simulink model "linear_simulation"  (R2022b)
settings: Solver=FixedStepAuto  StartTime=0.0  StopTime=10.0  FixedStep=1e-4  RelTol=1e-3  EnableMultiTasking=on
values from neighbouring files (symbols this model uses):
  beta = [0.5;2;2;0.5;1]    [Linear_optimal.m]
  delta = 1    [Linear_optimal.m]
  kl1 = sym2poly(kl1)    [Linear_optimal.m]
  kl2 = sym2poly(kl2)    [Linear_optimal.m]
  kn1 = sym2poly(kn1)    [Linear_optimal.m]
  kn2 = sym2poly(kn2)    [Linear_optimal.m]
libraries: simulink x6
settings Model: Creator=sf  LastModifiedBy=sf
settings ModelReferenceCC: EnableRefExpFcnMdlSchedulingChecks=on

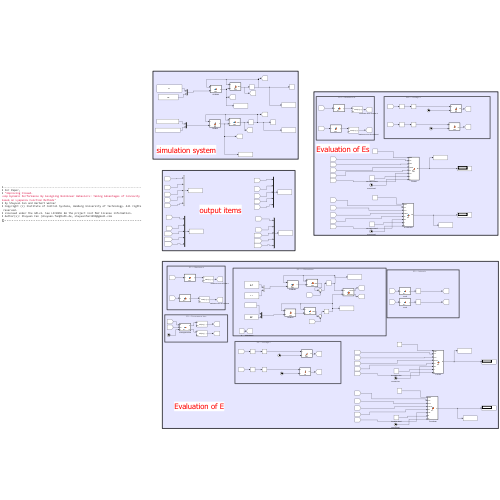
[thumbnail: Simulink's stored preview of the top-level diagram]
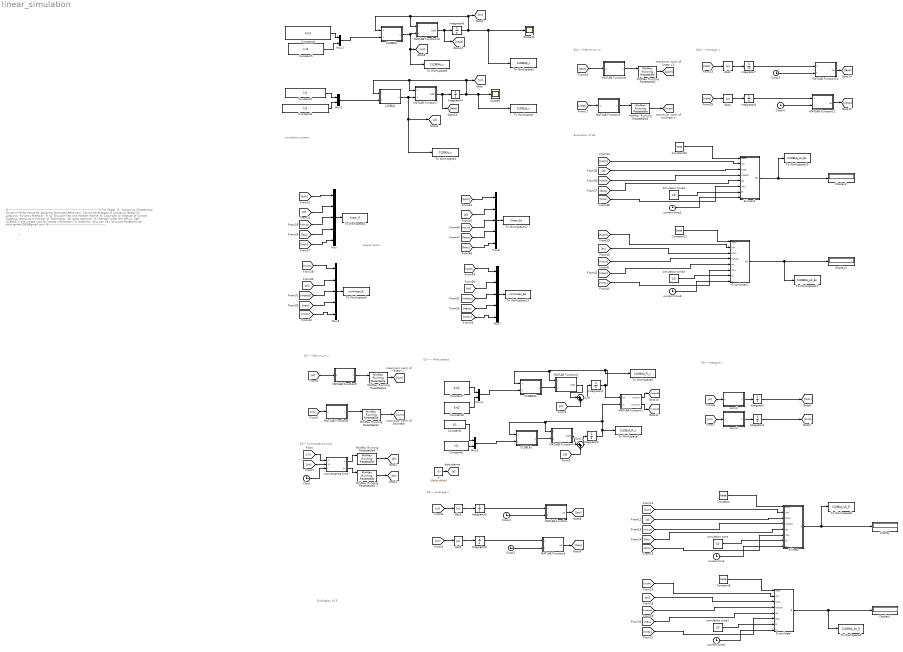
== system linear_simulation ==
  note: )
  note: %-----------------------------------------------------------------------------------------
      | % For Paper,
      | % "Improving Closed-Loop Dynamic Performance By Assigning Nonlinear Behaviors: Taking Advantages of Concavity Based on Lyapunov Function Methods"
      | % by Shuyuan Fan and Herbert Werner
      | % Copyright (c) Institute of Control Systems, Hamburg University of Technology. All rights reserved.
      | % Licensed under the GPLv3. See LICENSE in the project root for license information.
      | % Author(s): Shuyuan Fan (shuyuan.fan@tuhh.de, shuyuanfan1993@gmail.com
      | %---------------------------------------------------------
  note: Evaluation of E
  note: E5-----Integral x
  note: E3-------Robustness
  note: E1-----Maximum u
  note: E2----Convergence time
  note: E4-----everage u
  note: Es1-----Maximum us
  note: Es4-----everage u
  note: Evaluation of Es
  note: simulation system
  note: output items
  Abs{1..4} (4 alike) : Abs  SaturateOnIntegerOverflow=off
  CLDBLA : MATLAB Function  TreatAsAtomicUnit=on
  CLDBLA1 : MATLAB Function  TreatAsAtomicUnit=on
  CLDBNA : MATLAB Function  TreatAsAtomicUnit=on
  CLDBNA1 : MATLAB Function  TreatAsAtomicUnit=on
  Clock{,1..4} (5 alike) : Clock
  Constant{,9..11} (4 alike) : Constant  Value=beta
  Constant1 : Constant  Value=kl1
  Constant2 : Constant  Value=kl1
  Constant3 : Constant  Value=kl2
  Constant4 : Constant  Value=kn1
  Constant5 : Constant  Value=kn2
  Constant6 : Constant  Value=kl2
  Constant7 : Constant  Value=kn1
  Constant8 : Constant  Value=kn2
  Display{,1..3} (4 alike) : Display
  E-linear : MATLAB Function  TreatAsAtomicUnit=on
  E-linear1 : MATLAB Function  TreatAsAtomicUnit=on
  E-nonlinear : MATLAB Function  TreatAsAtomicUnit=on
  E-nonlinear1 : MATLAB Function  TreatAsAtomicUnit=on
  Integrator{,1,5..7,9} (6 alike) : Integrator
  Integrator{2..4,8} (4 alike) : Integrator  InitialCondition=[2;1]
  MATLAB Function : MATLAB Function  TreatAsAtomicUnit=on
  MATLAB Function1 : MATLAB Function  TreatAsAtomicUnit=on
  MATLAB Function10 : MATLAB Function  TreatAsAtomicUnit=on
  MATLAB Function11 : MATLAB Function  TreatAsAtomicUnit=on
  MATLAB Function13 : MATLAB Function  TreatAsAtomicUnit=on
  MATLAB Function2 : MATLAB Function  TreatAsAtomicUnit=on
  MATLAB Function3 : MATLAB Function  TreatAsAtomicUnit=on
  MATLAB Function4 : MATLAB Function  TreatAsAtomicUnit=on
  MATLAB Function5 : MATLAB Function  TreatAsAtomicUnit=on
  MATLAB Function6 : MATLAB Function  TreatAsAtomicUnit=on
  MATLAB Function7 : MATLAB Function  TreatAsAtomicUnit=on
  MATLAB Function8 : MATLAB Function  TreatAsAtomicUnit=on
  MATLAB Function9 : MATLAB Function  TreatAsAtomicUnit=on
  MinMax Running Resettable{1..3,7} (4 alike) : simulink/Math Operations/MinMax Running Resettable  Function=max  vinit=0.0
  MinMax Running Resettable4 : simulink/Math Operations/MinMax Running Resettable  Function=min  vinit=100
  MinMax Running Resettable5 : simulink/Math Operations/MinMax Running Resettable  Function=min  vinit=100
  Mux{,5..7} (4 alike) : Mux  Inputs=5
  Mux{1..4} (4 alike) : Mux  Inputs=2
  Scope11 : Scope
  Scope6 : Scope
  Sum : Sum  Inputs=|++
  Sum1 : Sum  Inputs=|++
  To Workspace : ToWorkspace  VariableName=CLDBLA_x  SaveFormat=Timeseries  SampleTime=-1
  To Workspace1 : ToWorkspace  VariableName=CLDBNA_x  SaveFormat=Timeseries  SampleTime=-1
  To Workspace10 : ToWorkspace  VariableName=CLDBLA_ob_Es  SaveFormat=Timeseries  SampleTime=-1
  To Workspace11 : ToWorkspace  VariableName=CLDBNA_ob_Es  SaveFormat=Timeseries  SampleTime=-1
  To Workspace12 : ToWorkspace  VariableName=linear_Es  SaveFormat=Timeseries  SampleTime=-1
  To Workspace13 : ToWorkspace  VariableName=nonlinear_Es  SaveFormat=Timeseries  SampleTime=-1
  To Workspace2 : ToWorkspace  VariableName=linear_E  SaveFormat=Timeseries  SampleTime=-1
  To Workspace3 : ToWorkspace  VariableName=nonlinear_E  SaveFormat=Timeseries  SampleTime=-1
  To Workspace4 : ToWorkspace  VariableName=CLDBLA_u  SaveFormat=Timeseries  SampleTime=-1
  To Workspace5 : ToWorkspace  VariableName=CLDBNA_u  SaveFormat=Timeseries  SampleTime=-1
  To Workspace6 : ToWorkspace  VariableName=CLDBNA_R_x  SaveFormat=Timeseries  SampleTime=-1
  To Workspace7 : ToWorkspace  VariableName=CLDBLA_R_x  SaveFormat=Timeseries  SampleTime=-1
  To Workspace8 : ToWorkspace  VariableName=CLDBLA_ob_E  SaveFormat=Timeseries  SampleTime=-1
  To Workspace9 : ToWorkspace  VariableName=CLDBNA_ob_E  SaveFormat=Timeseries  SampleTime=-1
  convergence time : MATLAB Function  TreatAsAtomicUnit=on
  current time{,1..3} (4 alike) : Clock
  d : Constant  Value=[delta;delta]
  norm2 : MATLAB Function  TreatAsAtomicUnit=on
  norm3 : MATLAB Function  TreatAsAtomicUnit=on
  simulation time{,1..3} (4 alike) : Constant  Value=10
  wires:
  Constant5/1 -> Mux2/2
  MATLAB Function7/1(xdot) -> [ldot], Integrator4/1
  Constant2/1 -> Mux1/1
  CLDBLA/1(u) -> To Workspace4/1, [ul], MATLAB Function7/2(u)
  Mux1/1 -> CLDBLA/2(k)
  Constant3/1 -> Mux1/2
  Mux2/1 -> CLDBNA/2(k)
  Constant4/1 -> Mux2/1
  MATLAB Function13/1(xdot) -> [ndot], Integrator8/1
  Integrator8/1 -> To Workspace1/1, Scope11/1, [xn], CLDBNA/1(x), MATLAB Function13/1(x)
  MATLAB Function5/1(y) -> MinMax Running Resettable1/1
  CLDBNA/1(u) -> To Workspace5/1, [un], MATLAB Function13/2(u)
  MinMax Running Resettable1/1 -> [lum]
  Clock/1 -> convergence time/3(t)
  Integrator4/1 -> To Workspace/1, Scope6/1, [xl], CLDBLA/1(x), MATLAB Function7/1(x)
  [xl] -> convergence time/1(xl)
  [xn] -> convergence time/2(xn)
  convergence time/1(tl) -> MinMax Running Resettable4/1
  convergence time/2(tn) -> MinMax Running Resettable5/1
  MinMax Running Resettable4/1 -> [tl]
  MinMax Running Resettable5/1 -> [tn]
  MATLAB Function2/1(xdot) -> Sum/1
  Mux4/1 -> CLDBNA1/2(k)
  Constant7/1 -> Mux4/1
  CLDBNA1/1(u) -> MATLAB Function2/2(u)
  CLDBLA1/1(u) -> MATLAB Function4/2(u)
  Constant6/1 -> Mux3/2
  Mux3/1 -> CLDBLA1/2(k)
  Constant8/1 -> Mux4/2
  Integrator3/1 -> MATLAB Function1/1(xn), To Workspace6/1, CLDBNA1/1(x), MATLAB Function2/1(x)
  Constant1/1 -> Mux3/1
  Integrator2/1 -> MATLAB Function1/2(xl), CLDBLA1/1(x), MATLAB Function4/1(x), To Workspace7/1
  MATLAB Function4/1(xdot) -> Sum1/1
  Sum/1 -> Integrator3/1
  Sum1/1 -> Integrator2/1
  d/1 -> [d]
  [d] -> Sum/2
  [d] -> Sum1/2
  [ul] -> MATLAB Function5/1(u)
  [un] -> MATLAB Function6/1(u)
  MinMax Running Resettable7/1 -> [num]
  [xl] -> norm2/1(u)
  norm2/1(y) -> Integrator/1
  Integrator/1 -> [lintx]
  Integrator1/1 -> [nintx]
  norm3/1(y) -> Integrator1/1
  [xn] -> norm3/1(u)
  [un] -> Abs3/1
  [ul] -> Abs2/1
  Abs3/1 -> Integrator6/1
  Abs2/1 -> Integrator5/1
  Integrator5/1 -> MATLAB Function/1(u)
  Clock1/1 -> MATLAB Function/2(t)
  Clock2/1 -> MATLAB Function3/2(t)
  Integrator6/1 -> MATLAB Function3/1(u)
  MATLAB Function/1(ua) -> [lau]
  MATLAB Function3/1(ua) -> [nau]
  MATLAB Function1/1(normxl) -> [lrobust]
  MATLAB Function1/2(normxn) -> [nrobust]
  [lum] -> E-linear/2(um)
  [tl] -> E-linear/3(tcon)
  [lrobust] -> E-linear/4(robust)
  [lau] -> E-linear/5(au)
  [lintx] -> E-linear/6(intx)
  simulation time/1 -> E-linear/7(tf)
  current time/1 -> E-linear/8(tc)
  Constant/1 -> E-linear/1(beta)
  E-linear/1(E) -> To Workspace8/1, Display/1
  [nrobust] -> E-nonlinear/4(robust)
  E-nonlinear/1(E) -> To Workspace9/1, Display1/1
  current time1/1 -> E-nonlinear/8(tc)
  Constant9/1 -> E-nonlinear/1(beta)
  [num] -> E-nonlinear/2(um)
  simulation time1/1 -> E-nonlinear/7(tf)
  [tn] -> E-nonlinear/3(tcon)
  [nintx] -> E-nonlinear/6(intx)
  [nau] -> E-nonlinear/5(au)
  [lum] -> Mux/1
  [tl] -> Mux/2
  [lrobust] -> Mux/3
  [lau] -> Mux/4
  [lintx] -> Mux/5
  Mux/1 -> To Workspace2/1
  Mux5/1 -> To Workspace3/1
  [num] -> Mux5/1
  [tn] -> Mux5/2
  [nrobust] -> Mux5/3
  [nau] -> Mux5/4
  [nintx] -> Mux5/5
  MATLAB Function6/1(y) -> MinMax Running Resettable7/1
  [ndot] -> MATLAB Function9/1(u)
  [ldot] -> MATLAB Function8/1(u)
  MATLAB Function8/1(y) -> MinMax Running Resettable2/1
  MATLAB Function9/1(y) -> MinMax Running Resettable3/1
  MinMax Running Resettable3/1 -> [nusm]
  MinMax Running Resettable2/1 -> [lusm]
  Integrator9/1 -> MATLAB Function11/1(u)
  Clock3/1 -> MATLAB Function10/2(t)
  MATLAB Function11/1(ua) -> [naus]
  [ldot] -> Abs1/1
  Integrator7/1 -> MATLAB Function10/1(u)
  Clock4/1 -> MATLAB Function11/2(t)
  MATLAB Function10/1(ua) -> [laus]
  Abs1/1 -> Integrator7/1
  Abs4/1 -> Integrator9/1
  [ndot] -> Abs4/1
  E-nonlinear1/1(Es) -> To Workspace11/1, Display3/1
  simulation time3/1 -> E-nonlinear1/7(tf)
  [lintx] -> E-linear1/6(intx)
  [lrobust] -> E-linear1/4(robust)
  [naus] -> E-nonlinear1/5(au)
  simulation time2/1 -> E-linear1/7(tf)
  [tl] -> E-linear1/3(tcon)
  [nintx] -> E-nonlinear1/6(intx)
  Constant11/1 -> E-nonlinear1/1(beta)
  E-linear1/1(Es) -> To Workspace10/1, Display2/1
  [nusm] -> E-nonlinear1/2(um)
  current time2/1 -> E-linear1/8(tc)
  [nrobust] -> E-nonlinear1/4(robust)
  Constant10/1 -> E-linear1/1(beta)
  [lusm] -> E-linear1/2(um)
  [laus] -> E-linear1/5(au)
  current time3/1 -> E-nonlinear1/8(tc)
  [tn] -> E-nonlinear1/3(tcon)
  [tl] -> Mux6/2
  [tn] -> Mux7/2
  [nrobust] -> Mux7/3
  [lintx] -> Mux6/5
  [lrobust] -> Mux6/3
  [laus] -> Mux6/4
  [lusm] -> Mux6/1
  [nintx] -> Mux7/5
  [nusm] -> Mux7/1
  Mux7/1 -> To Workspace13/1
  Mux6/1 -> To Workspace12/1
  [naus] -> Mux7/4

== matlab function linear_simulation/MATLAB Function3 ==
  data: u input; ua output; t input
function ua = fcn(u,t)
u1=u(1);
u2 = u(2);
if t ==0
    ua1 =0;
    ua2 =0;
else
  ua1 = u1/t;
  ua2 = u2/t;
end
ua = [ua1;ua2];

== matlab function linear_simulation/MATLAB Function5 ==
  data: u input; y output
function y = fcn(u)

y =norm(u);

== matlab function linear_simulation/MATLAB Function13 ==
  data: x input; u input; xdot output
function xdot = fcn(x,u)

x1= x(1);
x2 = x(2);
u1 = u(1);
u2 = u(2);
x1dot = -x1+x2+u1+u2;
x2dot = -x1+x2+2*u1+u2;
xdot = [x1dot;x2dot];

== matlab function linear_simulation/CLDBNA ==
  data: x input; u output; k input
function u = fcn(x,k)
x1 = x(1);
x2 = x(2);
k1 = k(1);
k2 = k(2);
% for x1
a1 = 0.4;
b1 = 0.02;
r1 = 2;
c1 = 1;
d1 = 1;
f1 = k1*Fcr(x1,a1,b1,r1,c1,d1);

% for x2
a2 = 0.5;
b2 = 0.04;
r2 = 2;
c2 = 1;
d2 = 1;
e2 = x2-0.5*x1;
f2 = k2*Fcr(e2,a2,b2,r2,c2,d2);

u1 = 0.5*(-2*f2+f1-x2-1.5*x1);
u2 = -f1+0.5*x1-u1;
u = [u1;u2];
end



















function F = Fcr(x,a,b,r,c,d)
% a,b,c,d>0, x^r>0
% a>b concave function
% a<b convex function
% Fcr = (c*x^r+a)/(d*x^r+b)*x;
% calculate derivative derivative
F = (c*x^r+a)/(d*x^r+b)*x;
end

== matlab function linear_simulation/E-nonlinear ==
  data: beta input; um input; E output; tcon input; robust input; au input; intx input; tf input; tc input
function E = fcn(beta,um,tcon,robust,au,intx,tf,tc)
beta1 = beta(1);
beta2 = beta(2);
beta3 = beta(3);
beta4 = beta(4);
beta5 = beta(5);
unm = um;
if tc<0.9*tf
    E = 0;
else
   E =beta1*unm + beta2*tcon + beta3*robust + beta4*norm(au)*tc/(tcon) + beta5*intx;   
end

== matlab function linear_simulation/E-linear ==
  data: beta input; um input; E output; tcon input; robust input; au input; intx input; tf input; tc input
function E = fcn(beta,um,tcon,robust,au,intx,tf,tc)
beta1 = beta(1);
beta2 = beta(2);
beta3 = beta(3);
beta4 = beta(4);
beta5 = beta(5);
unm = um;
if tc<0.9*tf
    E = 0;
else
   E =beta1*unm + beta2*tcon + beta3*robust + beta4*norm(au)*tc/(tcon) + beta5*intx;   
end

== matlab function linear_simulation/CLDBLA1 ==
  data: x input; u output; k input
function u = fcn(x,k)
x1 = x(1);
x2 = x(2);
k1 = k(1);
k2 = k(2);
% for x1
f1 = k1*x1;

% for x2
e2 = x2-0.5*x1;
f2 = k2*e2;

u1 = 0.5*(-2*f2+f1-x2-1.5*x1);
u2 = -f1+0.5*x1-u1;
u = [u1;u2];
end

== matlab function linear_simulation/MATLAB Function6 ==
  data: u input; y output
function y = fcn(u)

y =norm(u);

== matlab function linear_simulation/MATLAB Function8 ==
  data: u input; y output
function y = fcn(u)

y =norm(u);

== matlab function linear_simulation/MATLAB Function9 ==
  data: u input; y output
function y = fcn(u)

y =norm(u);

== matlab function linear_simulation/MATLAB Function10 ==
  data: u input; ua output; t input
function ua = fcn(u,t)
u1=u(1);
u2 = u(2);
if t ==0
    ua1 =0;
    ua2 =0;
else
  ua1 = u1/t;
  ua2 = u2/t;
end
ua = [ua1;ua2];

== matlab function linear_simulation/MATLAB Function11 ==
  data: u input; ua output; t input
function ua = fcn(u,t)
u1=u(1);
u2 = u(2);
if t ==0
    ua1 =0;
    ua2 =0;
else
  ua1 = u1/t;
  ua2 = u2/t;
end
ua = [ua1;ua2];

== matlab function linear_simulation/E-linear1 ==
  data: beta input; um input; Es output; tcon input; robust input; au input; intx input; tf input; tc input
function Es = fcn(beta,um,tcon,robust,au,intx,tf,tc)
beta1 = beta(1);
beta2 = beta(2);
beta3 = beta(3);
beta4 = beta(4);
beta5 = beta(5);
unm = um;
if tc<0.9*tf
    Es = 0;
else
   Es =beta1*unm + beta2*tcon + beta3*robust + beta4*norm(au)*tc/(tcon) + beta5*intx;   
end

== matlab function linear_simulation/E-nonlinear1 ==
  data: beta input; um input; Es output; tcon input; robust input; au input; intx input; tf input; tc input
function Es = fcn(beta,um,tcon,robust,au,intx,tf,tc)
beta1 = beta(1);
beta2 = beta(2);
beta3 = beta(3);
beta4 = beta(4);
beta5 = beta(5);
unm = um;
if tc<0.9*tf
    Es = 0;
else
   Es =beta1*unm + beta2*tcon + beta3*robust + beta4*norm(au)*tc/(tcon) + beta5*intx;   
end

== matlab function linear_simulation/convergence time ==
  data: xl input; tl output; xn input; t input; tn output
function [tl,tn] = fcn(xl,xn,t)

if norm(xl)<0.001
    tl = t;
else
    tl = 10000;
end
if norm(xn)<0.001
    tn = t;
else
    tn = 10000;
end

== matlab function linear_simulation/CLDBNA1 ==
  data: x input; u output; k input
function u = fcn(x,k)
x1 = x(1);
x2 = x(2);
k1 = k(1);
k2 = k(2);
% for x1
a1 = 0.4;
b1 = 0.02;
r1 = 2;
c1 = 1;
d1 = 1;
f1 = k1*Fcr(x1,a1,b1,r1,c1,d1);

% for x2
a2 = 0.5;
b2 = 0.04;
r2 = 2;
c2 = 1;
d2 = 1;
e2 = x2-0.5*x1;
f2 = k2*Fcr(e2,a2,b2,r2,c2,d2);

u1 = 0.5*(-2*f2+f1-x2-1.5*x1);
u2 = -f1+0.5*x1-u1;
u = [u1;u2];
end



















function F = Fcr(x,a,b,r,c,d)
% a,b,c,d>0, x^r>0
% a>b concave function
% a<b convex function
% Fcr = (c*x^r+a)/(d*x^r+b)*x;
% calculate derivative derivative
F = (c*x^r+a)/(d*x^r+b)*x;
end

== matlab function linear_simulation/MATLAB Function1 ==
  data: xn input; xl input; normxl output; normxn output
function [normxl,normxn]= fcn(xn,xl)
normxl = norm(xl);
normxn = norm(xn);

== matlab function linear_simulation/MATLAB Function2 ==
  data: x input; u input; xdot output
function xdot = fcn(x,u)

x1= x(1);
x2 = x(2);
u1 = u(1);
u2 = u(2);
x1dot = -x1+x2+u1+u2;
x2dot = -x1+x2+2*u1+u2;
xdot = [x1dot;x2dot];

== matlab function linear_simulation/norm2 ==
  data: u input; y output
function y = fcn(u)

y = norm(u);

== matlab function linear_simulation/MATLAB Function4 ==
  data: x input; u input; xdot output
function xdot = fcn(x,u)

x1= x(1);
x2 = x(2);
u1 = u(1);
u2 = u(2);
x1dot = -x1+x2+u1+u2;
x2dot = -x1+x2+2*u1+u2;
xdot = [x1dot;x2dot];

== matlab function linear_simulation/MATLAB Function ==
  data: u input; ua output; t input
function ua = fcn(u,t)
u1=u(1);
u2 = u(2);
if t ==0
    ua1 =0;
    ua2 =0;
else
  ua1 = u1/t;
  ua2 = u2/t;
end
ua = [ua1;ua2];

== matlab function linear_simulation/MATLAB Function7 ==
  data: x input; u input; xdot output
function xdot = fcn(x,u)

x1= x(1);
x2 = x(2);
u1 = u(1);
u2 = u(2);
x1dot = -x1+x2+u1+u2;
x2dot = -x1+x2+2*u1+u2;
xdot = [x1dot;x2dot];

== matlab function linear_simulation/CLDBLA ==
  data: x input; u output; k input
function u = fcn(x,k)
x1 = x(1);
x2 = x(2);
k1 = k(1);
k2 = k(2);
% for x1
f1 = k1*x1;

% for x2
e2 = x2-0.5*x1;
f2 = k2*e2;

u1 = 0.5*(-2*f2+f1-x2-1.5*x1);
u2 = -f1+0.5*x1-u1;
u = [u1;u2];
end

== matlab function linear_simulation/norm3 ==
  data: u input; y output
function y = fcn(u)

y = norm(u);
